simulink model "Lecture8_LoopDelay"  (R2020b)
settings: Solver=VariableStepAuto  StartTime=0.0  StopTime=10.0  RelTol=1e-3
values from neighbouring files (symbols this model uses):
  delay = (-pi/2)/(-wc)    (= 0.157079632679)    [Lecture8_LoopDelay.m]
settings Model: Creator=sebastian  LastModifiedBy=sebastian

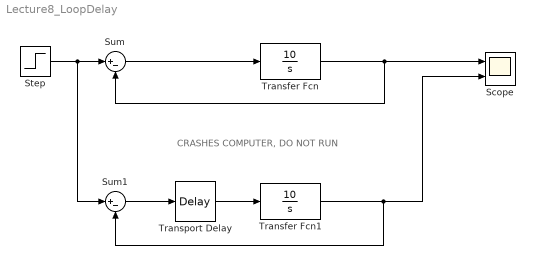
== system Lecture8_LoopDelay ==
  note: CRASHES COMPUTER, DO NOT RUN
  Scope : Scope  NumInputPorts=2
  Step : Step  SampleTime=0
  Sum : Sum  Inputs=|+-
  Sum1 : Sum  Inputs=|+-
  Transfer Fcn : TransferFcn  Numerator=[10]  Denominator=[1 0]
  Transfer Fcn1 : TransferFcn  Numerator=[10]  Denominator=[1 0]
  Transport Delay : TransportDelay  DelayTime=delay
  wires:
  Step/1 -> Sum1/1, Sum/1
  Sum/1 -> Transfer Fcn/1
  Sum1/1 -> Transport Delay/1
  Transport Delay/1 -> Transfer Fcn1/1
  Transfer Fcn/1 -> Sum/2, Scope/1
  Transfer Fcn1/1 -> Scope/2, Sum1/2
